simulink model "gm_HDLExampleFIL_vs"  (R2022b)
settings: Solver=FixedStepDiscrete  StartTime=0.0  StopTime=simTime  RelTol=1e-3
values from neighbouring files (symbols this model uses):
  sampleTime = 1    [exampleFIL.m]
libraries: simulink x2, dspsrcs4 x1, vivadosimlib x1
settings Model: Creator=cotti  LastModifiedBy=cotti
settings OptimizationCC: BlockReduction=off  ConditionallyExecuteInputs=off  DefaultParameterBehavior=Inlined  InheritOutputTypeSmallerThanSingle=on
settings DebuggingCC: AlgebraicLoopMsg=error  InheritedTsInSrcMsg=none  SingleTaskRateTransMsg=error
settings HardwareCC: ProdBitPerPointer=32  ProdBitPerSizeT=32  ProdBitPerPtrDiffT=32  ProdLargestAtomicFloat=None  ProdIntDivRoundTo=Undefined  ProdEndianess=Unspecified  ProdWordSize=32  ProdHWDeviceType=ASIC/FPGA->ASIC/FPGA  TargetBitPerLong=64  TargetBitPerPointer=64  TargetBitPerSizeT=64  TargetBitPerPtrDiffT=64  TargetLongLongMode=on  TargetIntDivRoundTo=Zero  TargetEndianess=LittleEndian  TargetWordSize=64  TargetHWDeviceType=Custom Processor->MATLAB Host Computer  ProdEqTarget=off

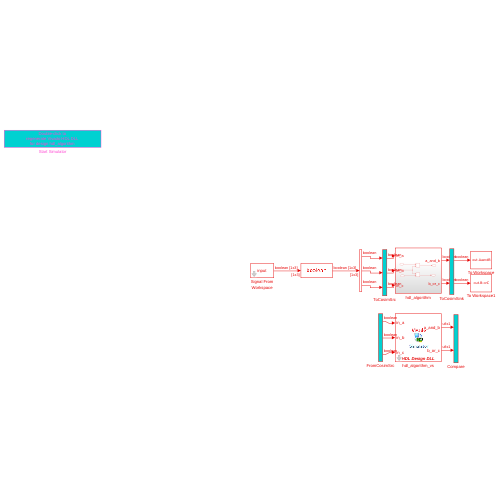
[thumbnail: Simulink's stored preview of the top-level diagram]
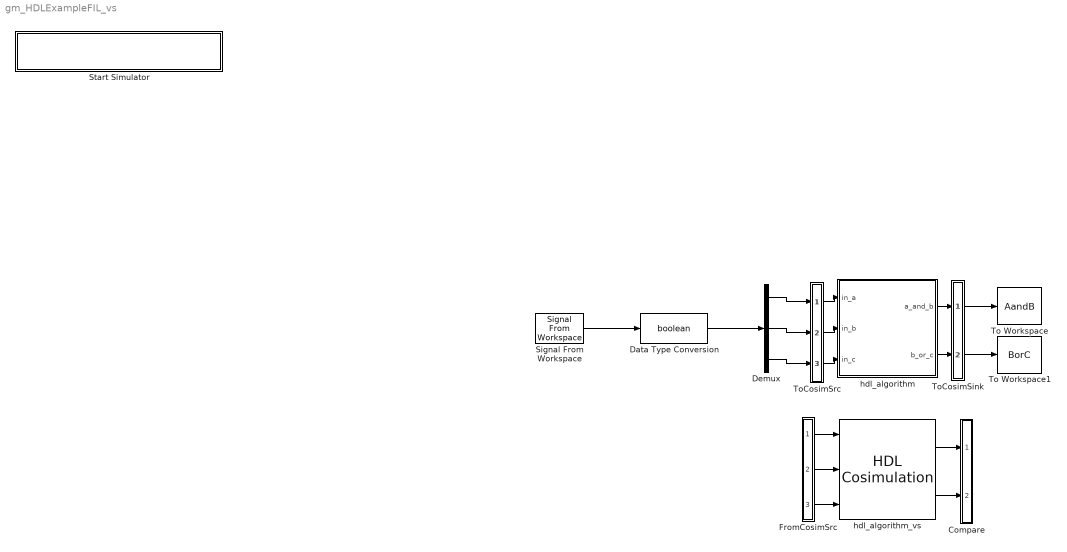
== system gm_HDLExampleFIL_vs ==
  Compare : Subsystem
      mask Display: disp('')
  Data Type Conversion : DataTypeConversion  OutDataTypeStr=boolean  SaturateOnIntegerOverflow=off  RndMeth=Floor
  Demux : Demux  Outputs=3
  FromCosimSrc : Subsystem
      mask Display: disp('')
  Signal From Workspace : dspsrcs4/Signal From Workspace  X=input  Ts=sampleTime  nsamps=sampleSize  OutputAfterFinalValue=Setting to zero  ignoreOrWarnInputAndFrameLengths=off  OutputFrames=off
  Start Simulator : Subsystem
      settings: OpenFcn=|
      | cosimDirName = pwd;
      | cd 'hdl_prj/hdlsrc/HDLExampleFIL';
      | [s,r] = system('vivado -mode batch -source gm_HDLExampleFIL_vs.tcl','-echo');
      | cd (cosimDirName);
      | clear cosimDirName;
      | if s
      |    error('Failed to create Vivado HDL design DLL using script gm_HDLExampleFIL_vs.tcl.');
      | end
      mask Display: disp('Double-click to\nregenerate Vivado HDL DLL\nfor design hdl_algorithm')
  To Workspace : ToWorkspace  VariableName=AandB  SaveFormat=Timeseries  SampleTime=-1
      settings: Save2DSignal=2-D array (concatenate along first dimension)
  To Workspace1 : ToWorkspace  VariableName=BorC  SaveFormat=Timeseries  SampleTime=-1
      settings: Save2DSignal=2-D array (concatenate along first dimension)
  ToCosimSink : Subsystem
      mask Display: disp('')
  ToCosimSrc : Subsystem
      mask Display: disp('')
  hdl_algorithm : Subsystem
  hdl_algorithm_vs : vivadosimlib/HDL Cosimulation  PortPaths=/hdl_algorithm/in_a;/hdl_algorithm/in_b;/hdl_algorithm/in_c;/hdl_algorithm/a_and_b;/hdl_algorithm/b_or_c  PortModes=[1 1 1 2 2 ]  PortTimes=[-1 -1 -1 1 1 ]  PortSigns=[-1 -1 -1 0 0 ]  PortFracLengths=[0,0,0,0,0]  CommLocal=on  CommSharedMemory=on  CommPortNumber=4449  CommShowInfo=on  ClockModes=[]  ClockTimes=[]  TclPostSimCommand="puts \"done\""  TimingMode=ns  TimingScaleFactor=10  idxCellArray={'UNUSED_VAR'}  CosimBypass=Full Simulation  AllowDirectFeedthrough=on  ProductName=EDA Simulator Link VS  RunAutoTimescale=off  HdlClocks=0  PreRunTime=0  PreRunTimeUnit=ns
  wires:
  Signal From Workspace/1 -> Data Type Conversion/1
  Data Type Conversion/1 -> Demux/1
  ToCosimSrc/1(out1) -> hdl_algorithm/1(in_a)
  ToCosimSrc/2(out2) -> hdl_algorithm/2(in_b)
  ToCosimSrc/3(out3) -> hdl_algorithm/3(in_c)
  hdl_algorithm/1(a_and_b) -> ToCosimSink/1(in1)
  hdl_algorithm/2(b_or_c) -> ToCosimSink/2(in2)
  Demux/1 -> ToCosimSrc/1(in1)
  Demux/2 -> ToCosimSrc/2(in2)
  Demux/3 -> ToCosimSrc/3(in3)
  ToCosimSink/1(out1) -> To Workspace/1
  ToCosimSink/2(out2) -> To Workspace1/1
  FromCosimSrc/1(out1) -> hdl_algorithm_vs/1
  FromCosimSrc/2(out2) -> hdl_algorithm_vs/2
  FromCosimSrc/3(out3) -> hdl_algorithm_vs/3
  hdl_algorithm_vs/1 -> Compare/1(in1)
  hdl_algorithm_vs/2 -> Compare/2(in2)

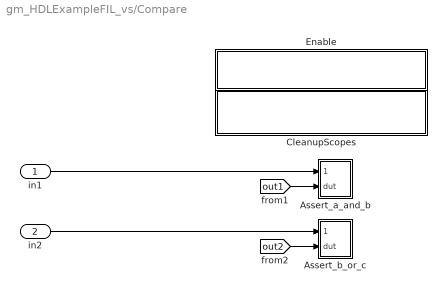
== system gm_HDLExampleFIL_vs/Compare ==
  in1 : Inport
  in2 : Inport  Port=2
  Assert_a_and_b : Subsystem
      settings: LibrarySourceBlock=hdlmdlgenlib/AssertEq
  Assert_b_or_c : Subsystem
      settings: LibrarySourceBlock=hdlmdlgenlib/AssertEq
  CleanupScopes : Subsystem
      settings: OpenFcn=|
      | blkName = gcb; %self block
      | idx = regexp(blkName, '/CleanupScopes$', 'once');
      | blkParent = blkName(1:idx-1);
      | blks=find_system(blkParent, 'LookUnderMasks', 'all','blocktype', 'Scope');
      | for itr = 1:length(blks)
      | 	 hScopeCfg = get_param(blks{itr},'ScopeConfiguration');
      | 	 hScopeCfg.Visible = ~ hScopeCfg.Visible;
      | end
      | drawnow;
      mask Display: fprintf(message('hdlcoder:cosim:vnl_dblclick').getString());
  Enable : Subsystem
      settings: OpenFcn=|
      | blkName = gcb;
      | idx = regexp(blkName, '/Enable$', 'once');
      | blkParent = blkName(1:idx-1);
      | blks=find_system(blkParent, 'LookUnderMasks', 'all','blocktype', 'Assertion');
      | e = get_param(blks{1}, 'Enabled');
      | if strcmp(e, 'on'), f= 'off';, else, f = 'on';, end
      | for ii=1:length(blks), set_param(blks{ii}, 'Enabled', f);, end
      | set_param(gcb, 'MaskDisplay',['fprintf(message(''hdlcoder:cosim:vnl_dblclick_assertions'',','''',upper(e),'''',').getString())']);
      mask Display: fprintf(message('hdlcoder:cosim:vnl_dblclick_assertions','OFF').getString());
  wires:
  in1/1 -> Assert_a_and_b/1(cosim)
  [out1] -> Assert_a_and_b/2(dut)
  in2/1 -> Assert_b_or_c/1(cosim)
  [out2] -> Assert_b_or_c/2(dut)

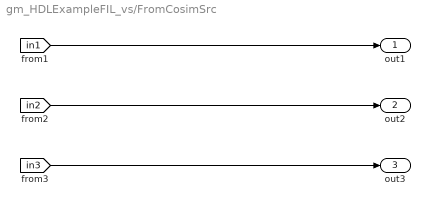
== system gm_HDLExampleFIL_vs/FromCosimSrc ==
  out1 : Outport
  out2 : Outport  Port=2
  out3 : Outport  Port=3
  wires:
  [in1] -> out1/1
  [in2] -> out2/1
  [in3] -> out3/1

== system gm_HDLExampleFIL_vs/Start Simulator ==

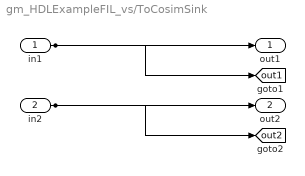
== system gm_HDLExampleFIL_vs/ToCosimSink ==
  in1 : Inport
  in2 : Inport  Port=2
  out1 : Outport
  out2 : Outport  Port=2
  tag scope: out1=global, out2=global
  wires:
  in1/1 -> out1/1, [out1]
  in2/1 -> out2/1, [out2]

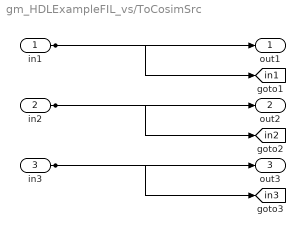
== system gm_HDLExampleFIL_vs/ToCosimSrc ==
  in1 : Inport
  in2 : Inport  Port=2
  in3 : Inport  Port=3
  out1 : Outport
  out2 : Outport  Port=2
  out3 : Outport  Port=3
  tag scope: in1=global, in2=global, in3=global
  wires:
  in1/1 -> out1/1, [in1]
  in2/1 -> out2/1, [in2]
  in3/1 -> out3/1, [in3]

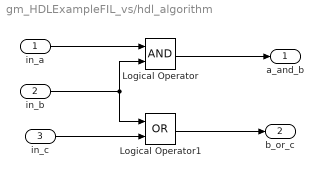
== system gm_HDLExampleFIL_vs/hdl_algorithm ==
  in_a : Inport
  in_b : Inport  Port=2
  in_c : Inport  Port=3
  Logical Operator : Logic  AllPortsSameDT=off  OutDataTypeStr=boolean
  Logical Operator1 : Logic  Operator=OR  AllPortsSameDT=off  OutDataTypeStr=boolean
  a_and_b : Outport
  b_or_c : Outport  Port=2
  wires:
  Logical Operator/1 -> a_and_b/1
  in_a/1 -> Logical Operator/1
  in_b/1 -> Logical Operator1/1, Logical Operator/2
  in_c/1 -> Logical Operator1/2
  Logical Operator1/1 -> b_or_c/1

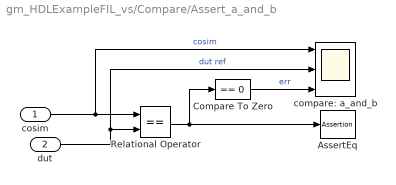
== system gm_HDLExampleFIL_vs/Compare/Assert_a_and_b ==
  cosim : Inport
  dut : Inport  Port=2
  AssertEq : Assertion
  Compare To Zero : simulink/Logic and Bit Operations/Compare To Zero  relop===  OutDataTypeStr=boolean
      settings: LibrarySourceBlock=|
      | hdlmdlgenlib/AssertEq/Compare
      | To Zero
  Relational Operator : RelationalOperator  Operator===  OutDataTypeStr=boolean  InputSameDT=off
  compare: a_and_b : Scope  NumInputPorts=3
  wires:
  Compare To Zero/1 -> compare: a_and_b/3  "err"
  Relational Operator/1 -> Compare To Zero/1, AssertEq/1
  cosim/1 -> compare: a_and_b/1, Relational Operator/1  "cosim"
  dut/1 -> compare: a_and_b/2, Relational Operator/2  "dut ref"

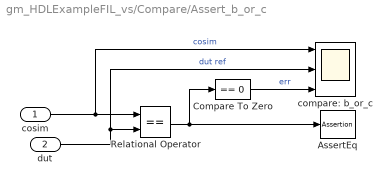
== system gm_HDLExampleFIL_vs/Compare/Assert_b_or_c ==
  cosim : Inport
  dut : Inport  Port=2
  AssertEq : Assertion
  Compare To Zero : simulink/Logic and Bit Operations/Compare To Zero  relop===  OutDataTypeStr=boolean
      settings: LibrarySourceBlock=|
      | hdlmdlgenlib/AssertEq/Compare
      | To Zero
  Relational Operator : RelationalOperator  Operator===  OutDataTypeStr=boolean  InputSameDT=off
  compare: b_or_c : Scope  NumInputPorts=3
  wires:
  Compare To Zero/1 -> compare: b_or_c/3  "err"
  Relational Operator/1 -> Compare To Zero/1, AssertEq/1
  cosim/1 -> compare: b_or_c/1, Relational Operator/1  "cosim"
  dut/1 -> compare: b_or_c/2, Relational Operator/2  "dut ref"

== system gm_HDLExampleFIL_vs/Compare/CleanupScopes ==

== system gm_HDLExampleFIL_vs/Compare/Enable ==
